simulink model "closed_loop_freq_todo"  (R2016b)
settings: Solver=VariableStepAuto  StartTime=0.0  StopTime=10.0  RelTol=1e-3
values from neighbouring files (symbols this model uses):
  Cs_den = cell2mat(Cs.Denominator)    [LCSproject.m]
  Cs_num = cell2mat(Cs.Numerator)    [LCSproject.m]
  delay_freq = 0.001    [LCSproject.m]
  tfPendDen = cell2mat(tfPend.Denominator)    [LCSproject.m]
  tfPendNum = cell2mat(tfPend.Numerator)    [LCSproject.m]
libraries: dspfdesign x1
settings Model: Creator=Olivier  LastModifiedBy=Olivier

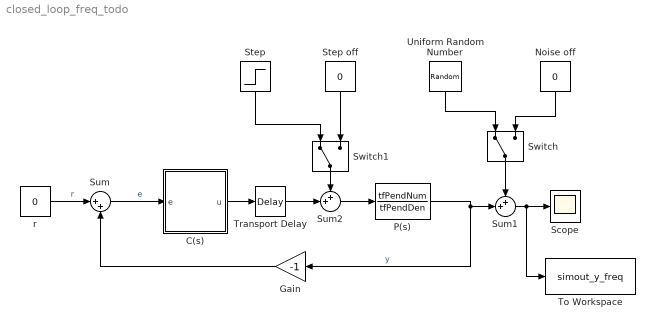
== system closed_loop_freq_todo ==
  C(s) : Subsystem
  Gain : Gain  Gain=-1
  Noise off : Constant  Value=0
  P(s) : TransferFcn  Numerator=tfPendNum  Denominator=tfPendDen
  Scope : Scope
  Step : Step  After=0.2  SampleTime=0
  Step off : Constant  Value=0
  Sum : Sum  Inputs=|++
  Sum1 : Sum  Inputs=++|
  Sum2 : Sum  Inputs=++|
  Switch : ManualSwitch
  Switch1 : ManualSwitch
  To Workspace : ToWorkspace  VariableName=simout_y_freq  SaveFormat=Timeseries  SampleTime=-1
  Transport Delay : TransportDelay  DelayTime=delay_freq
  Uniform Random Number : UniformRandomNumber  Minimum=-0.005  Maximum=0.005  SampleTime=0.1
  r : Constant  Value=0
  wires:
  r/1 -> Sum/1  "r"
  P(s)/1 -> Gain/1, Sum1/2  "y"
  Uniform Random Number/1 -> Switch/1
  Gain/1 -> Sum/2
  Transport Delay/1 -> Sum2/2
  Sum1/1 -> To Workspace/1, Scope/1
  Sum2/1 -> P(s)/1
  Step/1 -> Switch1/1
  Sum/1 -> C(s)/1(e)  "e"
  C(s)/1(u) -> Transport Delay/1
  Noise off/1 -> Switch/2
  Switch/1 -> Sum1/1
  Switch1/1 -> Sum2/1
  Step off/1 -> Switch1/2

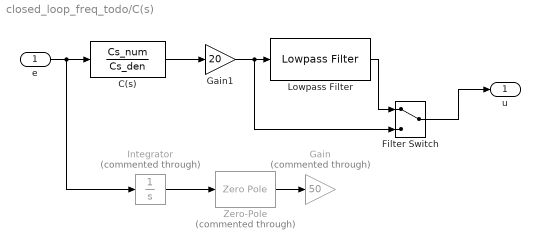
== system closed_loop_freq_todo/C(s) ==
  e : Inport
  C(s) : TransferFcn  Numerator=Cs_num  Denominator=Cs_den
  Filter Switch : ManualSwitch
  Gain : Gain  Commented=through  Gain=50
  Gain1 : Gain  Gain=20
  Integrator : Integrator  Commented=through
  Lowpass Filter : dspfdesign/Lowpass Filter  FilterType=FIR  DesignForMinimumOrder=on  FilterOrder=50  PassbandFrequency=8e3  StopbandFrequency=12e3  PassbandRipple=0.1  StopbandAttenuation=80  InheritSampleRate=off  SampleRate=44100  SimulateUsing=Interpreted execution  roundingMode=Floor  coeffsDataTypeStr=fixdt(1,16)
  Zero-Pole : ZeroPole  Commented=through  Poles=[0 -1]
  u : Outport
  wires:
  C(s)/1 -> Gain1/1
  Lowpass Filter/1 -> Filter Switch/1
  Filter Switch/1 -> u/1
  Zero-Pole/1 -> Gain/1
  Integrator/1 -> Zero-Pole/1
  e/1 -> Integrator/1, C(s)/1
  Gain1/1 -> Filter Switch/2, Lowpass Filter/1
